simulink model "w2_warplab_buffers"  (Simulink 7.7)
settings: Solver=VariableStepDiscrete  SolverMode=SingleTasking  StartTime=0.0  StopTime=200000  RelTol=1e-3
InitFcn:
  | w2_warplab_buffers_init
StartFcn:
  | w2_warplab_buffers_init
values from neighbouring files (symbols this model uses):
  NumSamps_Rx_IQ = 2^14    (= 16384)    [w2_warplab_buffers_init.m]
  NumSamps_Rx_RSSI = 2^12    (= 4096)    [w2_warplab_buffers_init.m]
  NumSamps_Tx_IQ = 2^14    (= 16384)    [w2_warplab_buffers_init.m]
undefined symbols (not defined in the file or in its folder): gcbh, xlBlockLoadCallback, xlGetNormalizedPeriod
libraries: xbsIndex_r4 x752
(part 7 of 7)

== system w2_warplab_buffers/Memory-mapped Registers/Timer64/usec Pulse ==
  Rst : Inport
  Clk->usec : xbsIndex_r4/Counter  cnt_type=Free Running  cnt_to=159  operation=Up  start_count=0  cnt_by_val=1  arith_type=Unsigned  n_bits=8  bin_pt=0  load_pin=off  rst=on  en=off  explicit_period=off  period=1  dbl_ovrd=off  use_behavioral_HDL=off  implementation=Fabric  block_type=counter
  Constant1 : xbsIndex_r4/Constant  const=39  gui_display_data_type=Fixed-point  arith_type=Unsigned  n_bits=8  bin_pt=0  preci_type=Single  exp_width=8  frac_width=24  explicit_period=off  period=1  equ=P=C  opselect=C  inp2=PCIN>>17  opr=+  inp1=P  carry=CIN  dbl_ovrd=off  block_type=constant
      settings: block_version=8.2.02
  Logical : xbsIndex_r4/Logical  logical_function=OR  inputs=2  en=off  latency=0  precision=Full  arith_type=Unsigned  n_bits=16  bin_pt=0  align_bp=on  dbl_ovrd=off  block_type=logical
  Relational : xbsIndex_r4/Relational  mode=a=b  en=off  latency=0  dbl_ovrd=off  block_type=relational
  uSec : Outport
  wires:
  Clk->usec/1 -> Relational/1
  Constant1/1 -> Relational/2
  Relational/1 -> uSec/1, Logical/1
  Logical/1 -> Clk->usec/1
  Rst/1 -> Logical/2
